simulink model "environmental_testing"  (R2019b)
settings: Solver=VariableStepAuto  StartTime=0.0  StopTime=11800  MaxStep=0.01  RelTol=1e-3
InitFcn:
  | Distance_travelled = [0: 1 :12000;0: 1 :12000;]';
settings Model: Creator=Avmash  LastModifiedBy=Avmash

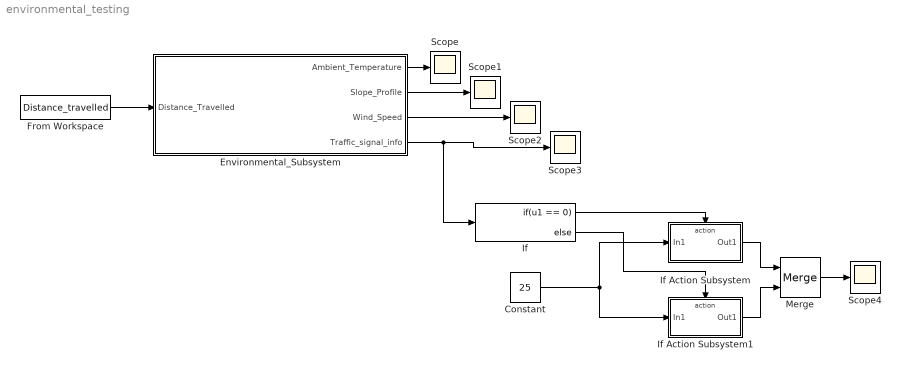
== system environmental_testing ==
  Constant : Constant  Value=25
  Environmental_Subsystem : Subsystem
  From Workspace : FromWorkspace  VariableName=Distance_travelled  SampleTime=0
  If : If  IfExpression=u1 == 0
  If Action Subsystem : Subsystem  TreatAsAtomicUnit=on
  If Action Subsystem1 : Subsystem  TreatAsAtomicUnit=on
  Merge : Merge
  Scope{,1..4} (5 alike) : Scope
  wires:
  Environmental_Subsystem/3(Wind_Speed) -> Scope2/1
  Environmental_Subsystem/2(Slope_Profile) -> Scope1/1
  Environmental_Subsystem/1(Ambient_Temperature) -> Scope/1
  From Workspace/1 -> Environmental_Subsystem/1(Distance_Travelled)
  Environmental_Subsystem/4(Traffic_signal_info) -> If/1, Scope3/1
  If/1 -> If Action Subsystem/Action
  If/2 -> If Action Subsystem1/Action
  Constant/1 -> If Action Subsystem1/1(In1), If Action Subsystem/1(In1)
  If Action Subsystem1/1(Out1) -> Merge/2
  If Action Subsystem/1(Out1) -> Merge/1
  Merge/1 -> Scope4/1

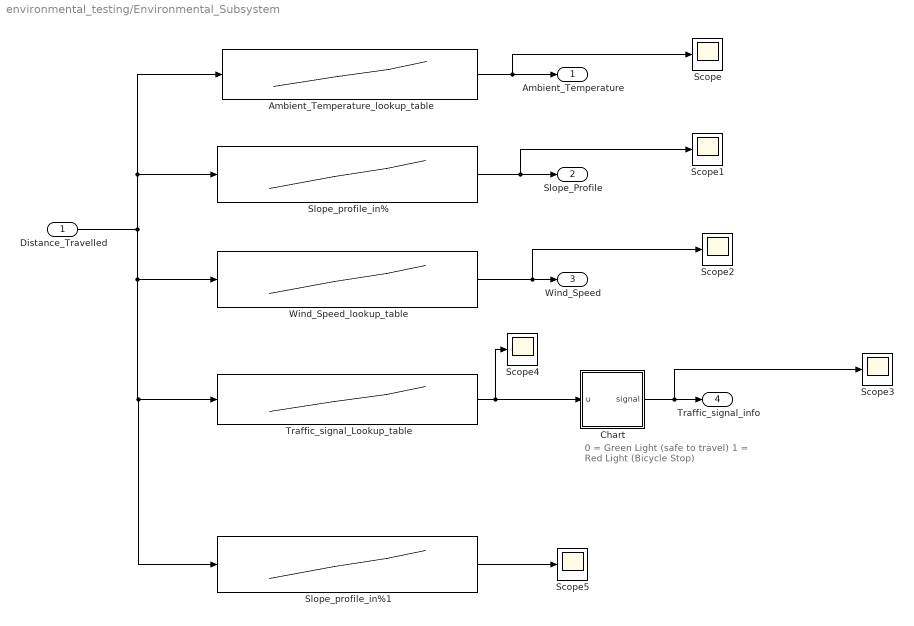
== system environmental_testing/Environmental_Subsystem ==
  note: 0 = Green Light (safe to travel)
      | 1 = Red Light (Bicycle Stop)
  Distance_Travelled : Inport
  Ambient_Temperature_lookup_table : Lookup_n-D  NumberOfTableDimensions=1  BreakpointsForDimension1=[0 6000 12000]  Table=[25 24 25]  InternalRulePriority=Speed  RndMeth=Simplest  InputSameDT=on
  Chart : Stateflow chart  BlockKeywords=__PRM__SERIALIZED__DATA__:Stateflow Chart,Stateflow Diagram  TreatAsAtomicUnit=on
  Scope{,1..5} (6 alike) : Scope
  Slope_profile_in% : Lookup_n-D  NumberOfTableDimensions=1  BreakpointsForDimension1=|  Table=|  InternalRulePriority=Speed  RndMeth=Simplest  InputSameDT=on
      BreakpointsForDimension1=|
      | [0000,
      | 0015,
      | 0056,
      | 0099,
      | 0108,
      | 0118,
      | 0132,
      | 0142,
      | 0160,
      | 0170,
      | 0186,
      | 0228,
      | 0293,
      | 0336,
      | 0363,
      | 0381,
      | 0391,
      | 0402,
      | 0437,
      | 0478,
      | 0538,
      | 0565,
      | 0582,
      | 0591,
      | 0611,
      | 0640,
      | 0675,
      | 0684,
      | 0699,
      | 0757,
      | 0777,
      | 0788,
      | 0820,
      | 0823,
      | 0837,
      | 0841,
      | 0863,
      | 0880,
      | 0900,
      | 0918,
      | 0948,
      | 0985,
      | 1016,
      | 1037,
      | 1051,
      | 1061,
      | 1082,
      | 1113,
      | 1134,
      | 1142,
      | 1151,
      | 1165,
      | 1176,
      | 1187,
      | 1200,
      | 1216,
      | 1234,
      | 1277,
      | 1341,
      | 1373,
      | 1401,
      | 1452,
      | 1486,
      | 1497,
      | 1507,
      | 1520,
      | 1528,
      | 1557,
      | 1649,
      | 1694,
      | 1716,
      | 1767,
      | 1827,
      | 1898,
      | 1946,
      | 2017,
      | 2030,
      | 2040,
      | 2056,
      | 2110,
      | 2201,
      | 2231,
      | 2242,
      | 2325,
      | 2412,
      | 2504,
      | 2530,
      | 2570,
      | 2607,
      | 2640,
      | 2665,
      | 2713,
      | 2730,
      | 2752,
      | 2763,
      | 2774,
      | 2863,
      | 2961,
      | 3095,
      | 3167,
      | 3268,
      | 3368,
      | 3384,
      | 3418,
      | 3480,
      | 3503,
      | 3562,
      | 3601,
      | 3635,
      | 3719,
      | 3748,
      | 3768,
      | 3844,
      | 3916,
      | 4078,
      | 4224,
      | 4305,
      | 4357,
      | 4398,
      | 4445,
      | 4493,
      | 4548,
      | 4641,
      | 4770,
      | 4916,
      | 5015,
      | 5084,
      | 5110,
      | 5212,
      | 5458,
      | 5491,
      | 5525,
      | 5541,
      | 5551,
      | 5562,
      | 5574,
      | 5591,
      | 5622,
      | 5652,
      | 5665,
      | 5727,
      | 5806,
      | 5856,
      | 5914,
      | 5974,
      | 6031,
      | 6097,
      | 6322,
      | 6482,
      | 6528,
      | 6632,
      | 6688,
      | 6763,
      | 6810,
      | 6853,
      | 6910,
      | 6951,
      | 6998,
      | 7051,
      | 7185,
      | 7248,
      | 7303,
      | 7349,
      | 7386,
      | 7421,
      | 7455,
      | 7492,
      | 7530,
      | 7567,
      | 7609,
      | 7691,
      | 7747,
      | 7751,
      | 7764,
      | 7775,
      | 7808,
      | 7833,
      | 8143,
      | 8170,
      | 8180,
      | 8210,
      | 8811,
      | 8980,
      | 9047,
      | 9065,
      | 9086,
      | 9104,
      | 9141,
      | 9168,
      | 9191,
      | 9215,
      | 9249,
      | 9296,
      | 9348,
      | 9405,
      | 9426,
      | 9442,
      | 9473,
      | 9515,
      | 9550,
      | 9581,
      | 9601,
      | 9627,
      | 9652,
      | 9682,
      | 9735,
      | 9760,
      | 9774,
      | 9784,
      | 9797,
      | 9818,
      | 9838,
      | 9858,
      | 9880,
      | 9972,
      | 10015,
      | 10110,
      | 10128,
      | 10180,
      | 10196,
      | 10262,
      | 10271,
      | 10295,
      | 10311,
      | 10379,
      | 10402,
      | 10421,
      | 10433,
      | 10449,
      | 10470,
      | 10483,
      | 10492,
      | 10501,
      | 10541,
      | 10561,
      | 10573,
      | 10601,
      | 10626,
      | 10652,
      | 10709,
      | 10748,
      | 10809,
      | 10840,
      | 10860,
      | 10877,
      | 10888,
      | 10897,
      | 10912,
      | 10927,
      | 10988,
      | 11013,
      | 11027,
      | 11042,
      | 11084,
      | 11094,
      | 11117,
      | 11138,
      | 11167,
      | 11197,
      | 11251,
      | 11270,
      | 11290,
      | 11304,
      | 11320,
      | 11335,
      | 11351,
      | 11367,
      | 11446,
      | 11492,
      | 11514,
      | 11529,
      | 11540,
      | 11579,
      | 11596,
      | 11645,
      | 11667,
      | 11674,
      | 11689,
      | 11702,
      | 11800
      | ]
      Table=|
      | [0,
      | -0.487804878,
      | -0.23255814,
      | 0,
      | -1,
      | 0,
      | 0,
      | 0,
      | 0,
      | 0,
      | -0.714285714,
      | -0.769230769,
      | -0.697674419,
      | -0.740740741,
      | 0,
      | 0,
      | 0,
      | -0.285714286,
      | -0.243902439,
      | -0.166666667,
      | -0.37037037,
      | -0.588235294,
      | 0,
      | 0,
      | 0,
      | 0,
      | 0,
      | 0,
      | -0.344827586,
      | 0,
      | 0,
      | -0.3125,
      | 0,
      | -0.714285714,
      | 0,
      | 0,
      | 0,
      | 0,
      | 0,
      | 0.333333333,
      | 0.27027027,
      | 0,
      | 0,
      | 0,
      | -1,
      | 0,
      | 0,
      | 0,
      | 0,
      | 0,
      | 0,
      | 0,
      | 0,
      | 0,
      | 0,
      | 0,
      | 0,
      | 0,
      | 0.3125,
      | 0,
      | 0,
      | 0,
      | 0,
      | 0,
      | 0,
      | 0,
      | 0.344827586,
      | 0,
      | 0,
      | 0,
      | 0,
      | 0,
      | 0,
      | 0,
      | 0,
      | 0,
      | 0,
      | 0,
      | -0.185185185,
      | 0,
      | 0,
      | 0,
      | 0,
      | 0,
      | 0,
      | 0,
      | 0,
      | 0,
      | 0,
      | 0,
      | 0,
      | 0.588235294,
      | 0,
      | 0,
      | 0,
      | -0.112359551,
      | 0,
      | 0,
      | 0,
      | 0,
      | 0.1,
      | 0,
      | 0,
      | 0,
      | -0.434782609,
      | -0.169491525,
      | 0,
      | 0,
      | 0,
      | 0,
      | 0,
      | 0,
      | 0,
      | -0.061728395,
      | 0,
      | 0,
      | 0,
      | 0,
      | 0,
      | 0,
      | 0,
      | 0,
      | 0,
      | 0,
      | 0,
      | 0,
      | 0,
      | 0,
      | 0,
      | 0.303030303,
      | 0,
      | 0.625,
      | 0,
      | 0,
      | 0.833333333,
      | 0,
      | 0.322580645,
      | 0,
      | 0,
      | -0.322580645,
      | -0.379746835,
      | 0,
      | 0,
      | 0,
      | 0.175438596,
      | 0,
      | 0,
      | 0,
      | 0,
      | -0.096153846,
      | 0,
      | -0.133333333,
      | 0.212765957,
      | 0,
      | 0,
      | 0,
      | 0.212765957,
      | 0,
      | 0,
      | 0,
      | 0,
      | 0.217391304,
      | 0,
      | 0,
      | 0,
      | 0,
      | 0,
      | 0,
      | 0.238095238,
      | 0.12195122,
      | 0.357142857,
      | 0,
      | 0,
      | 0,
      | 0,
      | 0.4,
      | 0,
      | 0,
      | 0,
      | 0.333333333,
      | 0,
      | 0,
      | 0.149253731,
      | 0,
      | 0,
      | 0,
      | 0,
      | -0.37037037,
      | 0,
      | -0.416666667,
      | 0,
      | -0.212765957,
      | -0.192307692,
      | -0.175438596,
      | 0,
      | 0,
      | 0,
      | -0.238095238,
      | -0.285714286,
      | 0,
      | 0.5,
      | 0.384615385,
      | 0.4,
      | 0,
      | 0,
      | 0,
      | 0,
      | 0,
      | 0,
      | 0,
      | 0,
      | 0,
      | 0,
      | 0,
      | 0,
      | 0,
      | 0,
      | 0.192307692,
      | 0,
      | 0,
      | 0,
      | 0,
      | 0,
      | 0,
      | 0,
      | 0,
      | 0,
      | 0,
      | 0,
      | 0,
      | 0,
      | 0,
      | 0,
      | 0.5,
      | 0,
      | 0,
      | 0,
      | 0,
      | 0,
      | 0,
      | 0,
      | 0,
      | 0,
      | -0.588235294,
      | 0,
      | 0,
      | 0,
      | 0,
      | 0,
      | 0,
      | 0,
      | 0,
      | 0,
      | 0,
      | 0,
      | 0,
      | 0,
      | 0,
      | 0,
      | 0,
      | 0,
      | 0,
      | 0.625,
      | 0,
      | 0,
      | 0,
      | -0.126582278,
      | 0,
      | 0,
      | 0,
      | 0,
      | 0,
      | 0,
      | 0,
      | 0,
      | 0,
      | 0,
      | 0,
      | 0,
      | 0,
      | ]
  Slope_profile_in%1 : Lookup_n-D  NumberOfTableDimensions=1  BreakpointsForDimension1=|  IndexSearchMethod=Linear search  Table=|  InternalRulePriority=Speed  RndMeth=Simplest  InputSameDT=on
      BreakpointsForDimension1=|
      | [0000,
      | 0015,
      | 0056,
      | 0099,
      | 0108,
      | 0118,
      | 0132,
      | 0142,
      | 0160,
      | 0170,
      | 0186,
      | 0228,
      | 0293,
      | 0336,
      | 0363,
      | 0381,
      | 0391,
      | 0402,
      | 0437,
      | 0478,
      | 0538,
      | 0565,
      | 0582,
      | 0591,
      | 0611,
      | 0640,
      | 0675,
      | 0684,
      | 0699,
      | 0757,
      | 0777,
      | 0788,
      | 0820,
      | 0823,
      | 0837,
      | 0841,
      | 0863,
      | 0880,
      | 0900,
      | 0918,
      | 0948,
      | 0985,
      | 1016,
      | 1037,
      | 1051,
      | 1061,
      | 1082,
      | 1113,
      | 1134,
      | 1142,
      | 1151,
      | 1165,
      | 1176,
      | 1187,
      | 1200,
      | 1216,
      | 1234,
      | 1277,
      | 1341,
      | 1373,
      | 1401,
      | 1452,
      | 1486,
      | 1497,
      | 1507,
      | 1520,
      | 1528,
      | 1557,
      | 1649,
      | 1694,
      | 1716,
      | 1767,
      | 1827,
      | 1898,
      | 1946,
      | 2017,
      | 2030,
      | 2040,
      | 2056,
      | 2110,
      | 2201,
      | 2231,
      | 2242,
      | 2325,
      | 2412,
      | 2504,
      | 2530,
      | 2570,
      | 2607,
      | 2640,
      | 2665,
      | 2713,
      | 2730,
      | 2752,
      | 2763,
      | 2774,
      | 2863,
      | 2961,
      | 3095,
      | 3167,
      | 3268,
      | 3368,
      | 3384,
      | 3418,
      | 3480,
      | 3503,
      | 3562,
      | 3601,
      | 3635,
      | 3719,
      | 3748,
      | 3768,
      | 3844,
      | 3916,
      | 4078,
      | 4224,
      | 4305,
      | 4357,
      | 4398,
      | 4445,
      | 4493,
      | 4548,
      | 4641,
      | 4770,
      | 4916,
      | 5015,
      | 5084,
      | 5110,
      | 5212,
      | 5458,
      | 5491,
      | 5525,
      | 5541,
      | 5551,
      | 5562,
      | 5574,
      | 5591,
      | 5622,
      | 5652,
      | 5665,
      | 5727,
      | 5806,
      | 5856,
      | 5914,
      | 5974,
      | 6031,
      | 6097,
      | 6322,
      | 6482,
      | 6528,
      | 6632,
      | 6688,
      | 6763,
      | 6810,
      | 6853,
      | 6910,
      | 6951,
      | 6998,
      | 7051,
      | 7185,
      | 7248,
      | 7303,
      | 7349,
      | 7386,
      | 7421,
      | 7455,
      | 7492,
      | 7530,
      | 7567,
      | 7609,
      | 7691,
      | 7747,
      | 7751,
      | 7764,
      | 7775,
      | 7808,
      | 7833,
      | 8143,
      | 8170,
      | 8180,
      | 8210,
      | 8811,
      | 8980,
      | 9047,
      | 9065,
      | 9086,
      | 9104,
      | 9141,
      | 9168,
      | 9191,
      | 9215,
      | 9249,
      | 9296,
      | 9348,
      | 9405,
      | 9426,
      | 9442,
      | 9473,
      | 9515,
      | 9550,
      | 9581,
      | 9601,
      | 9627,
      | 9652,
      | 9682,
      | 9735,
      | 9760,
      | 9774,
      | 9784,
      | 9797,
      | 9818,
      | 9838,
      | 9858,
      | 9880,
      | 9972,
      | 10015,
      | 10110,
      | 10128,
      | 10180,
      | 10196,
      | 10262,
      | 10271,
      | 10295,
      | 10311,
      | 10379,
      | 10402,
      | 10421,
      | 10433,
      | 10449,
      | 10470,
      | 10483,
      | 10492,
      | 10501,
      | 10541,
      | 10561,
      | 10573,
      | 10601,
      | 10626,
      | 10652,
      | 10709,
      | 10748,
      | 10809,
      | 10840,
      | 10860,
      | 10877,
      | 10888,
      | 10897,
      | 10912,
      | 10927,
      | 10988,
      | 11013,
      | 11027,
      | 11042,
      | 11084,
      | 11094,
      | 11117,
      | 11138,
      | 11167,
      | 11197,
      | 11251,
      | 11270,
      | 11290,
      | 11304,
      | 11320,
      | 11335,
      | 11351,
      | 11367,
      | 11446,
      | 11492,
      | 11514,
      | 11529,
      | 11540,
      | 11579,
      | 11596,
      | 11645,
      | 11667,
      | 11674,
      | 11689,
      | 11702,
      | 11800
      | ]
      Table=|
      | [39,
      | 39,
      | 37,
      | 36,
      | 36,
      | 35,
      | 35,
      | 35,
      | 35,
      | 35,
      | 35,
      | 32,
      | 27,
      | 24,
      | 22,
      | 22,
      | 22,
      | 22,
      | 21,
      | 20,
      | 19,
      | 18,
      | 17,
      | 17,
      | 17,
      | 17,
      | 17,
      | 17,
      | 17,
      | 15,
      | 15,
      | 15,
      | 14,
      | 14,
      | 13,
      | 13,
      | 13,
      | 13,
      | 13,
      | 13,
      | 14,
      | 15,
      | 15,
      | 15,
      | 15,
      | 14,
      | 14,
      | 14,
      | 14,
      | 14,
      | 14,
      | 14,
      | 14,
      | 14,
      | 14,
      | 14,
      | 14,
      | 14,
      | 14,
      | 15,
      | 15,
      | 15,
      | 15,
      | 15,
      | 15,
      | 15,
      | 15,
      | 16,
      | 16,
      | 16,
      | 16,
      | 16,
      | 16,
      | 16,
      | 16,
      | 16,
      | 16,
      | 16,
      | 16,
      | 15,
      | 15,
      | 15,
      | 15,
      | 15,
      | 15,
      | 15,
      | 15,
      | 15,
      | 15,
      | 15,
      | 15,
      | 15,
      | 16,
      | 16,
      | 16,
      | 16,
      | 15,
      | 15,
      | 15,
      | 15,
      | 15,
      | 16,
      | 16,
      | 16,
      | 16,
      | 15,
      | 14,
      | 14,
      | 14,
      | 14,
      | 14,
      | 14,
      | 14,
      | 14,
      | 13,
      | 13,
      | 13,
      | 13,
      | 13,
      | 13,
      | 13,
      | 13,
      | 13,
      | 13,
      | 13,
      | 13,
      | 13,
      | 13,
      | 13,
      | 13,
      | 14,
      | 14,
      | 15,
      | 15,
      | 15,
      | 16,
      | 16,
      | 17,
      | 17,
      | 17,
      | 15,
      | 12,
      | 12,
      | 12,
      | 12,
      | 13,
      | 13,
      | 13,
      | 13,
      | 13,
      | 12,
      | 12,
      | 11,
      | 12,
      | 12,
      | 12,
      | 12,
      | 13,
      | 13,
      | 13,
      | 13,
      | 13,
      | 14,
      | 14,
      | 14,
      | 14,
      | 14,
      | 14,
      | 14,
      | 15,
      | 16,
      | 18,
      | 18,
      | 18,
      | 18,
      | 18,
      | 19,
      | 19,
      | 19,
      | 19,
      | 20,
      | 20,
      | 20,
      | 21,
      | 21,
      | 21,
      | 21,
      | 21,
      | 20,
      | 20,
      | 19,
      | 19,
      | 18,
      | 17,
      | 16,
      | 16,
      | 16,
      | 16,
      | 15,
      | 14,
      | 14,
      | 15,
      | 16,
      | 17,
      | 17,
      | 17,
      | 17,
      | 17,
      | 17,
      | 17,
      | 17,
      | 17,
      | 17,
      | 17,
      | 17,
      | 17,
      | 17,
      | 17,
      | 18,
      | 18,
      | 18,
      | 18,
      | 18,
      | 18,
      | 18,
      | 18,
      | 18,
      | 18,
      | 18,
      | 18,
      | 18,
      | 18,
      | 18,
      | 18,
      | 19,
      | 19,
      | 19,
      | 19,
      | 19,
      | 19,
      | 19,
      | 19,
      | 19,
      | 19,
      | 18,
      | 18,
      | 18,
      | 18,
      | 18,
      | 18,
      | 18,
      | 18,
      | 18,
      | 18,
      | 18,
      | 18,
      | 18,
      | 18,
      | 18,
      | 18,
      | 18,
      | 18,
      | 18,
      | 19,
      | 19,
      | 19,
      | 19,
      | 18,
      | 18,
      | 18,
      | 18,
      | 18,
      | 18,
      | 18,
      | 18,
      | 18,
      | 18,
      | 18,
      | 18,
      | 18
      | ]
  Traffic_signal_Lookup_table : Lookup_n-D  NumberOfTableDimensions=1  BreakpointsForDimension1=|  Table=|  InternalRulePriority=Speed  RndMeth=Simplest  InputSameDT=on
      BreakpointsForDimension1=|
      | [0,
      | 1352.604,
      | 1352.624,
      | 1352.644,
      | 2594.125,
      | 2594.145,
      | 2594.165,
      | 5283.812,
      | 5283.832,
      | 5283.852,
      | 7423.782,
      | 7423.802,
      | 7423.822,
      | 9090.133,
      | 9090.153,
      | 9090.173,
      | 9442.834,
      | 9442.854,
      | 9442.874,
      | 9911.784,
      | 9911.804,
      | 9911.824,
      | 10337.11,
      | 10337.31,
      | 10337.51,
      | 10698.74,
      | 10698.94,
      | 10699.14,
      | 11070.92,
      | 11071.12,
      | 11071.32,
      | 11082.84,
      | 11083.04,
      | 11083.24,
      | 11800
      | ]
      Table=|
      | [
      | 0,
      | 0,
      | 1,
      | 0,
      | 0,
      | 1,
      | 0,
      | 0,
      | 1,
      | 0,
      | 0,
      | 1,
      | 0,
      | 0,
      | 1,
      | 0,
      | 0,
      | 1,
      | 0,
      | 0,
      | 1,
      | 0,
      | 0,
      | 1,
      | 0,
      | 0,
      | 1,
      | 0,
      | 0,
      | 1,
      | 0,
      | 0,
      | 1,
      | 0,
      | 0]
  Wind_Speed_lookup_table : Lookup_n-D  NumberOfTableDimensions=1  BreakpointsForDimension1=[0 5999.9 6000 12000]  Table=[17 17 -17 -17]  InternalRulePriority=Speed  RndMeth=Simplest  InputSameDT=on
  Ambient_Temperature : Outport  VectorParamsAs1DForOutWhenUnconnected=off
  Slope_Profile : Outport  Port=2  VectorParamsAs1DForOutWhenUnconnected=off
  Wind_Speed : Outport  Port=3  VectorParamsAs1DForOutWhenUnconnected=off
  Traffic_signal_info : Outport  Port=4  VectorParamsAs1DForOutWhenUnconnected=off
  wires:
  Distance_Travelled/1 -> Wind_Speed_lookup_table/1, Slope_profile_in%1/1, Traffic_signal_Lookup_table/1, Slope_profile_in%/1, Ambient_Temperature_lookup_table/1
  Wind_Speed_lookup_table/1 -> Scope2/1, Wind_Speed/1
  Ambient_Temperature_lookup_table/1 -> Ambient_Temperature/1, Scope/1
  Slope_profile_in%/1 -> Slope_Profile/1, Scope1/1
  Chart/1(signal) -> Scope3/1, Traffic_signal_info/1
  Traffic_signal_Lookup_table/1 -> Chart/1(u), Scope4/1
  Slope_profile_in%1/1 -> Scope5/1

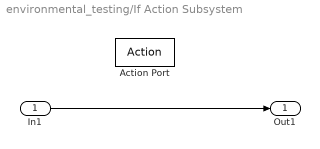
== system environmental_testing/If Action Subsystem ==
  In1 : Inport
  Action Port : ActionPort  ActionPortLabel=if(u1 == 0)
  Out1 : Outport
  wires:
  In1/1 -> Out1/1

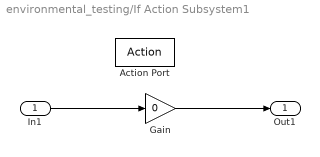
== system environmental_testing/If Action Subsystem1 ==
  In1 : Inport
  Action Port : ActionPort  ActionPortLabel=else
  Gain : Gain  Gain=0
  Out1 : Outport
  wires:
  In1/1 -> Gain/1
  Gain/1 -> Out1/1

== stateflow chart environmental_testing/Environmental_Subsystem/Chart ==
  (junction 5) -> (junction 9) : {signal=1}
  (junction 2) -> (junction 5) [order 1] : [u>0]
  (junction 9) -> (junction 15)
  (default) -> (junction 2)
  (junction 15) -> (junction 18)
  (junction 2) -> (junction 7) [order 2] : [u==0]
  (junction 13) -> (junction 15)
  (junction 7) -> (junction 13) : {signal=0}
  data: u input; signal output
